simulink library "cbc"  (Simulink 8.1)
settings: Solver=ode1  StartTime=0.0  StopTime=Inf  FixedStep=0.001  RelTol=1e-3
PostLoadFcn:
  | , if any(exist('dsrtsu_mdlpostloadfcn', 'file') == [2, 3, 6]), try dsrtsu_mdlpostloadfcn('Execute', bdroot); catch fprintf('Error in PostLoadFcn (dsrtsu_mdlpostloadfcn) for model "%s":\n %s\n', bdroot, lasterr); end, end,
libraries: dec x1, dlw x1, drr x1
settings Model: DSRTSU_INTERNAL_RTI_VER=450  DSRTSU_INTERNAL_RTI_TYPE=rti1401  RTICANMMDATA=struct('GeneralSetupData',struct('modelroot','D:\ELN150201_TAIWAN\trunk\AdasDragon\software\sw_development\arch\app\acc','generalsettings',struct('filesettings',struct('destfolder',struct('Name','RTICANMM_FILES','Check',1),'buildfolder',struct('Name','.','Check',1),'AbsDestfolder',struct('Name','D:\ELN150201_TAIWAN\trunk\AdasDragon\software\sw_development\arch\app\acc\RTICANMM_FILES'),'AbsBuildfolder',struct('Name','D:\ELN150201_TAIWAN\trunk\AdasDragon\software\sw_development\arch\app\acc'))),'options',struct('addpaths',1,'rmpaths',1,'addtrcexclusion',logical(1),'cannavigator',struct('checkmonitoring',0),'show_usrtrc',0,'use_usrtrc',0),'advanced',struct('options',[1 1 1 1 1 1 1 1 1 1 1 1 1 1 1 1 1 1 1 1 1 1 1 1 1 1 1 1 1 1 1 1 1 1 1 1 1 1 1 1 1 1 1 1 1 1 1 1 1 1 1 1 1 1 1 1 1 1 1 1 1 1 1 1 1 1 1 1 1 1 1 1 1 1 1 1 1 1 1 1 1 1 1 1 1 1 1 1 1 1 1 1 1 1 1 1 1 1 1 1]),'MPSetup',{{}},'modelname','cbc','block','cbc'))  DSRTSU_INTERNAL_RTIFPGA=40  Creator=tescamilla  LastModifiedBy=AT015555

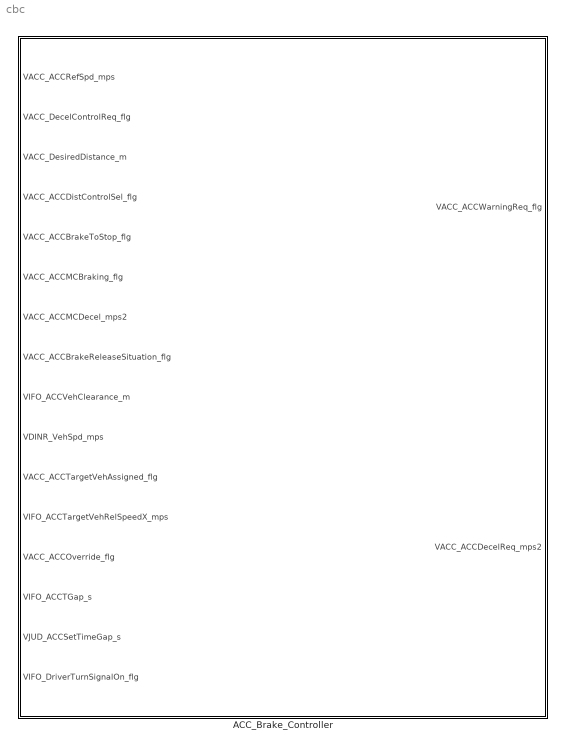
== system cbc ==
  ACC_Brake_Controller : Subsystem

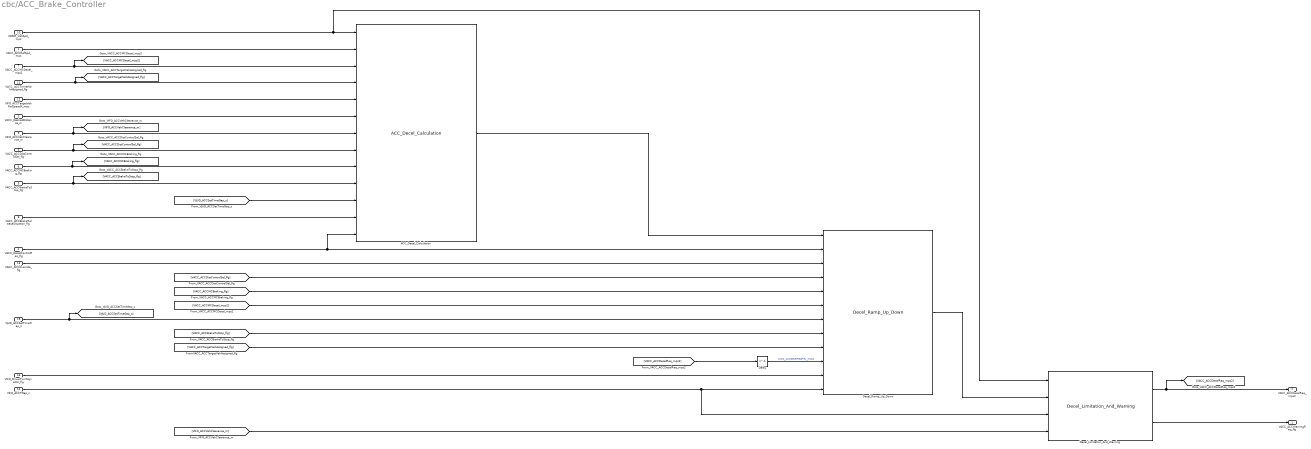
== system cbc/ACC_Brake_Controller ==
  VACC_ACCRefSpd_mps : Inport
  VACC_DecelControlReq_flg : Inport  Port=2
  VACC_DesiredDistance_m : Inport  Port=3
  VACC_ACCDistControlSel_flg : Inport  Port=4
  VACC_ACCBrakeToStop_flg : Inport  Port=5
  VACC_ACCMCBraking_flg : Inport  Port=6
  VACC_ACCMCDecel_mps2 : Inport  Port=7
  VACC_ACCBrakeReleaseSituation_flg : Inport  Port=8
  VIFO_ACCVehClearance_m : Inport  Port=9
  VDINR_VehSpd_mps : Inport  Port=10
  VACC_ACCTargetVehAssigned_flg : Inport  Port=11
  VIFO_ACCTargetVehRelSpeedX_mps : Inport  Port=12
  VACC_ACCOverride_flg : Inport  Port=13
  VIFO_ACCTGap_s : Inport  Port=14
  VJUD_ACCSetTimeGap_s : Inport  Port=15
  VIFO_DriverTurnSignalOn_flg : Inport  Port=16
  ACC_Decel_Calculation : dec/ACC_Decel_Calculation
  Decel_Limitation_And_Warning : dlw/Decel_Limitation_And_Warning
  Decel_Ramp_Up_Down : drr/Decel_Ramp_Up_Down
  Delay : Delay  DelayLength=1  InitialCondition=0
  VACC_ACCWarningReq_flg : Outport
  VACC_ACCDecelReq_mps2 : Outport  Port=2
  wires:
  Decel_Limitation_And_Warning/2 -> VACC_ACCWarningReq_flg/1
  Decel_Limitation_And_Warning/1 -> [VACC_ACCDecelReq_mps2], VACC_ACCDecelReq_mps2/1
  VDINR_VehSpd_mps/1 -> Decel_Limitation_And_Warning/1, ACC_Decel_Calculation/1
  Decel_Ramp_Up_Down/1 -> Decel_Limitation_And_Warning/2
  VACC_ACCOverride_flg/1 -> Decel_Ramp_Up_Down/3
  VACC_ACCRefSpd_mps/1 -> ACC_Decel_Calculation/2
  VACC_ACCMCDecel_mps2/1 -> [VACC_ACCMCDecel_mps2], ACC_Decel_Calculation/3
  VACC_ACCTargetVehAssigned_flg/1 -> [VACC_ACCTargetVehAssigned_flg], ACC_Decel_Calculation/4
  VIFO_ACCTargetVehRelSpeedX_mps/1 -> ACC_Decel_Calculation/5
  VACC_DesiredDistance_m/1 -> ACC_Decel_Calculation/6
  VACC_DecelControlReq_flg/1 -> ACC_Decel_Calculation/13, Decel_Ramp_Up_Down/2
  ACC_Decel_Calculation/1 -> Decel_Ramp_Up_Down/1
  VACC_ACCDistControlSel_flg/1 -> [VACC_ACCDistControlSel_flg], ACC_Decel_Calculation/8
  VACC_ACCMCBraking_flg/1 -> [VACC_ACCMCBraking_flg], ACC_Decel_Calculation/9
  [VACC_ACCDistControlSel_flg] -> Decel_Ramp_Up_Down/4
  VACC_ACCBrakeToStop_flg/1 -> [VACC_ACCBrakeToStop_flg], ACC_Decel_Calculation/10
  VIFO_ACCVehClearance_m/1 -> [VIFO_ACCVehClearance_m], ACC_Decel_Calculation/7
  [VIFO_ACCVehClearance_m] -> Decel_Limitation_And_Warning/4
  [VACC_ACCMCBraking_flg] -> Decel_Ramp_Up_Down/5
  [VACC_ACCMCDecel_mps2] -> Decel_Ramp_Up_Down/6
  VIFO_ACCTGap_s/1 -> Decel_Ramp_Up_Down/12, Decel_Limitation_And_Warning/3
  VJUD_ACCSetTimeGap_s/1 -> [VJUD_ACCSetTimeGap_s], Decel_Ramp_Up_Down/7
  [VJUD_ACCSetTimeGap_s] -> ACC_Decel_Calculation/11
  [VACC_ACCBrakeToStop_flg] -> Decel_Ramp_Up_Down/8
  [VACC_ACCTargetVehAssigned_flg] -> Decel_Ramp_Up_Down/9
  [VACC_ACCDecelReq_mps2] -> Delay/1
  Delay/1 -> Decel_Ramp_Up_Down/10  "VACC_ACCDecelReqPrev_mps2"
  VIFO_DriverTurnSignalOn_flg/1 -> Decel_Ramp_Up_Down/11
  VACC_ACCBrakeReleaseSituation_flg/1 -> ACC_Decel_Calculation/12
